simulink model "wcusp_bursting"  (Simulink 8.5)
settings: Solver=ode45  StartTime=0.0  StopTime=200  RelTol=1e-6
InitFcn:
  | wcusp_burst_params
values from neighbouring files (symbols this model uses):
  alpha = 0.7    [wcusp_burst_params.m]    (also in wcusp_params.m)
  beta = 0.5    [wcusp_burst_params.m]    (also in wcusp_params.m)
  delta = 1    [wcusp_burst_params.m]    (also in wcusp_params.m)
  k_u = 5    [wcusp_burst_params.m]
  tau_f = 0.0075    [wcusp_burst_params.m]    (also in wcusp_params.m)
  tau_s = 1    [wcusp_burst_params.m]    (also in wcusp_params.m)
  tau_u = 75    [wcusp_burst_params.m]
  x_u = 0.75    [wcusp_burst_params.m]
  xf_0 = -1    [wcusp_burst_params.m]    (also in wcusp_params.m)
  xs_0 = -1    [wcusp_burst_params.m]    (also in wcusp_params.m)
  xu_0 = -1    [wcusp_burst_params.m]
libraries: simulink x1
settings Model: Creator=tbb29  LastModifiedBy=ra428
settings DataIOCC: SignalLoggingSaveFormat=Dataset
settings OptimizationCC: ExpressionDepthLimit=128
settings DebuggingCC: UnderspecifiedInitializationDetection=Simplified  MergeDetectMultiDrivingBlocksExec=error  SolverPrmCheckMsg=warning  FcnCallInpInsideContextMsg=EnableAllAsWarning  StateNameClashWarn=none
settings GRTTargetCC: CombineOutputUpdateFcns=on  GRTInterface=off

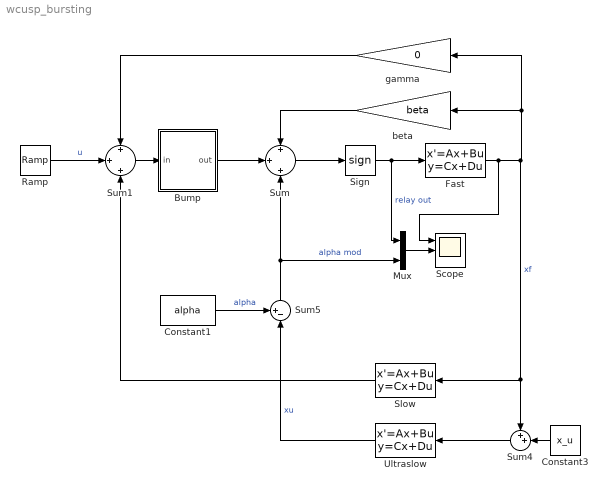
== system wcusp_bursting ==
  Bump : Subsystem
  Constant1 : Constant  Value=alpha
  Constant3 : Constant  Value=x_u
  Fast : StateSpace  A=-1/tau_f  B=1/tau_f  D=0  X0=xf_0
  Mux : Mux  Inputs=2
  Ramp : simulink/Sources/Ramp  slope=0  start=0  X0=0.5
  Scope : Scope  NumInputPorts=3
      settings: TimeRange=11.61971830985916  YMin=-2~-1~-1  YMax=2~2~1
  Sign : Signum
  Slow : StateSpace  A=-1/tau_s  B=1/tau_s  D=0  X0=xs_0
  Sum : Sum  Inputs=+|+|+
  Sum1 : Sum  Inputs=+|+|+
  Sum4 : Sum  Inputs=++|
  Sum5 : Sum  Inputs=+-|
  Ultraslow : StateSpace  A=-1/tau_u  B=k_u/tau_u  D=0  X0=xu_0
  beta : Gain  Gain=beta
  gamma : Gain  Gain=0
  wires:
  Sum/1 -> Sign/1
  beta/1 -> Sum/1
  Sign/1 -> Mux/1, Fast/1  "relay out"
  Fast/1 -> beta/1, gamma/1, Slow/1, Sum4/1, Scope/1  "xf"
  Sum1/1 -> Bump/1(in)
  Slow/1 -> Sum1/3
  gamma/1 -> Sum1/1
  Sum4/1 -> Ultraslow/1
  Constant3/1 -> Sum4/2
  Constant1/1 -> Sum5/1  "alpha"
  Sum5/1 -> Mux/2, Sum/3  "alpha mod"
  Ultraslow/1 -> Sum5/2  "xu"
  Bump/1(out) -> Sum/2
  Ramp/1 -> Sum1/2  "u"
  Mux/1 -> Scope/2

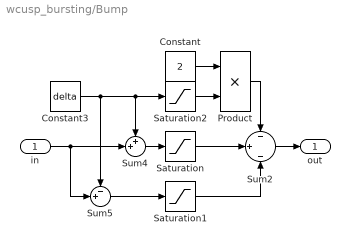
== system wcusp_bursting/Bump ==
  in : Inport
  Constant : Constant  Value=2
  Constant3 : Constant  Value=delta
  Product : Product  RndMeth=Zero
  Saturation : Saturate  UpperLimit=1  LowerLimit=-1
  Saturation1 : Saturate  UpperLimit=1  LowerLimit=-1
  Saturation2 : Saturate  UpperLimit=1  LowerLimit=-1
  Sum2 : Sum  Inputs=-|+|-
  Sum4 : Sum  Inputs=++|
  Sum5 : Sum  Inputs=-+|
  out : Outport
  wires:
  Saturation1/1 -> Sum2/3
  Saturation/1 -> Sum2/2
  Product/1 -> Sum2/1
  Saturation2/1 -> Product/2
  Constant/1 -> Product/1
  Constant3/1 -> Saturation2/1, Sum4/1, Sum5/1
  Sum4/1 -> Saturation/1
  in/1 -> Sum5/2, Sum4/2
  Sum5/1 -> Saturation1/1
  Sum2/1 -> out/1
